simulink subsystem "patient_state_to_bus"  (R2020b)
settings: Solver=VariableStepAuto  StartTime=0.0  StopTime=10.0  RelTol=1e-3
settings Model: Creator=RH  LastModifiedBy=Marco

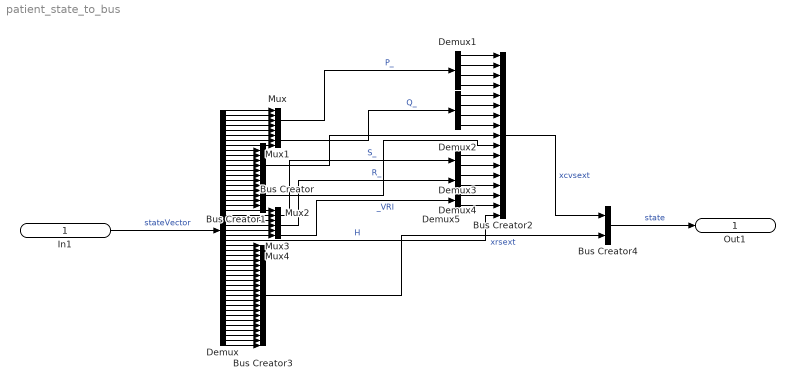
== system patient_state_to_bus ==
  In1 : Inport  PortDimensions=48
  Bus Creator : BusCreator  Inputs=6  OutDataTypeStr=Bus: ventricleInfo
      settings: InheritFromInputs=off
  Bus Creator1 : BusCreator  Inputs=6  OutDataTypeStr=Bus: ventricleInfo
      settings: InheritFromInputs=off
  Bus Creator2 : BusCreator  Inputs=17  OutDataTypeStr=Bus: CardioVascularStateExtended
      settings: InheritFromInputs=off
  Bus Creator3 : BusCreator  Inputs=21  OutDataTypeStr=Bus: RespiratoryStateExtended
      settings: InheritFromInputs=off
  Bus Creator4 : BusCreator  Inputs=2  OutDataTypeStr=Bus: PatientState
      settings: InheritFromInputs=off
  Demux : Demux  Outputs=48
  Demux1 : Demux
  Demux2 : Demux
  Demux3 : Demux  Outputs=2
  Demux4 : Demux  Outputs=2
  Demux5 : Demux  Outputs=2
  Mux : Mux
  Mux1 : Mux
  Mux2 : Mux  Inputs=2
  Mux3 : Mux  Inputs=2
  Mux4 : Mux  Inputs=2
  Out1 : Outport  OutDataTypeStr=Bus: PatientState
  wires:
  Demux/9 -> Bus Creator/1
  Demux1/4 -> Bus Creator2/4
  Demux/20 -> Bus Creator1/6
  Demux/12 -> Bus Creator/4
  Demux/7 -> Mux1/3
  Demux2/1 -> Bus Creator2/5
  Demux/43 -> Bus Creator3/16
  Bus Creator3/1 -> Bus Creator4/2  "xrsext"
  Demux/11 -> Bus Creator/3
  Demux3/1 -> Bus Creator2/11
  Demux/31 -> Bus Creator3/4
  Demux/1 -> Mux/1
  Demux/24 -> Mux3/2
  Demux/13 -> Bus Creator/5
  Demux/42 -> Bus Creator3/15
  Demux5/1 -> Bus Creator2/15
  Demux/4 -> Mux/4
  Demux/22 -> Mux2/2
  Demux3/2 -> Bus Creator2/12
  Demux/28 -> Bus Creator3/1
  Demux1/1 -> Bus Creator2/1
  Demux/21 -> Mux2/1
  Demux/32 -> Bus Creator3/5
  Demux/16 -> Bus Creator1/2
  Demux/8 -> Mux1/4
  Demux/25 -> Mux4/1
  Demux4/1 -> Bus Creator2/13
  Demux/36 -> Bus Creator3/9
  Demux/17 -> Bus Creator1/3
  Demux/5 -> Mux1/1
  Bus Creator/1 -> Bus Creator2/9
  Demux/27 -> Bus Creator2/17  "H"
  Demux/19 -> Bus Creator1/5
  Demux/39 -> Bus Creator3/12
  Demux/33 -> Bus Creator3/6
  Demux/44 -> Bus Creator3/17
  Demux1/2 -> Bus Creator2/2
  Bus Creator2/1 -> Bus Creator4/1  "xcvsext"
  Mux/1 -> Demux1/1  "P_"
  Demux5/2 -> Bus Creator2/16
  Demux/46 -> Bus Creator3/19
  Mux2/1 -> Demux3/1  "S_"
  Demux4/2 -> Bus Creator2/14
  Demux2/2 -> Bus Creator2/6
  Demux/40 -> Bus Creator3/13
  Mux3/1 -> Demux4/1  "R_"
  Demux/14 -> Bus Creator/6
  Demux/47 -> Bus Creator3/20
  Demux/18 -> Bus Creator1/4
  Demux/34 -> Bus Creator3/7
  Demux/23 -> Mux3/1
  Bus Creator1/1 -> Bus Creator2/10
  Demux/48 -> Bus Creator3/21
  Mux1/1 -> Demux2/1  "Q_"
  Demux2/4 -> Bus Creator2/8
  Mux4/1 -> Demux5/1  "_VRI"
  Demux/37 -> Bus Creator3/10
  Demux2/3 -> Bus Creator2/7
  Demux/41 -> Bus Creator3/14
  Demux/38 -> Bus Creator3/11
  Demux/3 -> Mux/3
  Demux/30 -> Bus Creator3/3
  Demux/2 -> Mux/2
  Demux1/3 -> Bus Creator2/3
  Demux/35 -> Bus Creator3/8
  Demux/6 -> Mux1/2
  Demux/29 -> Bus Creator3/2
  Demux/26 -> Mux4/2
  Demux/45 -> Bus Creator3/18
  Demux/15 -> Bus Creator1/1
  Demux/10 -> Bus Creator/2
  In1/1 -> Demux/1  "stateVector"
  Bus Creator4/1 -> Out1/1  "state"
